simulink model "state_space_obs"  (R2021a)
settings: Solver=VariableStepAuto  StartTime=0.0  StopTime=10.0  RelTol=1e-3
values from neighbouring files (symbols this model uses):
  A = [2 3;-1 4]    [simple_obs_deign.m]
  Aobs = [A-L*C]    [simple_obs_deign.m]
  B = [0;1]    [simple_obs_deign.m]
  Bobs = [B L]    [simple_obs_deign.m]
  C = [1 0]    [simple_obs_deign.m]
  Cobs = eye(2)    [simple_obs_deign.m]
settings Model: Creator=dfcpstage6  LastModifiedBy=dfcpstage6

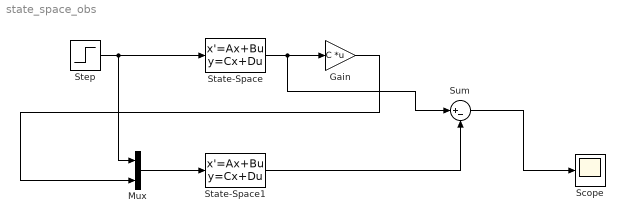
== system state_space_obs ==
  Gain : Gain  Gain=C  Multiplication=Matrix(K*u)
  Mux : Mux  Inputs=2
  Scope : Scope
  State-Space : StateSpace  A=A  B=B  C=eye(2)  D=zeros(2,1)  InitialCondition=0
  State-Space1 : StateSpace  A=Aobs  B=Bobs  C=Cobs  D=zeros(2,2)  InitialCondition=[0.01;0.01]
  Step : Step  SampleTime=0
  Sum : Sum  Inputs=|+-
  wires:
  Step/1 -> Mux/1, State-Space/1
  Mux/1 -> State-Space1/1
  State-Space/1 -> Sum/1, Gain/1
  Gain/1 -> Mux/2
  Sum/1 -> Scope/1
  State-Space1/1 -> Sum/2
